simulink model "RobustControl"  (Simulink 7.9)
settings: Solver=ode45  StartTime=0.0  StopTime=10.0  RelTol=1e-3
undefined symbols (not defined in the file): e, kd1, kd2, kd3, kd4, kd5, kd6, kp1, kp2, kp3, kp4, kp5, kp6, LinePTs2Rpm, PosSourceSelect, r, Ts
libraries: powerlib_extras x3
settings Model: Creator=Administrator  LastModifiedBy=Administrator

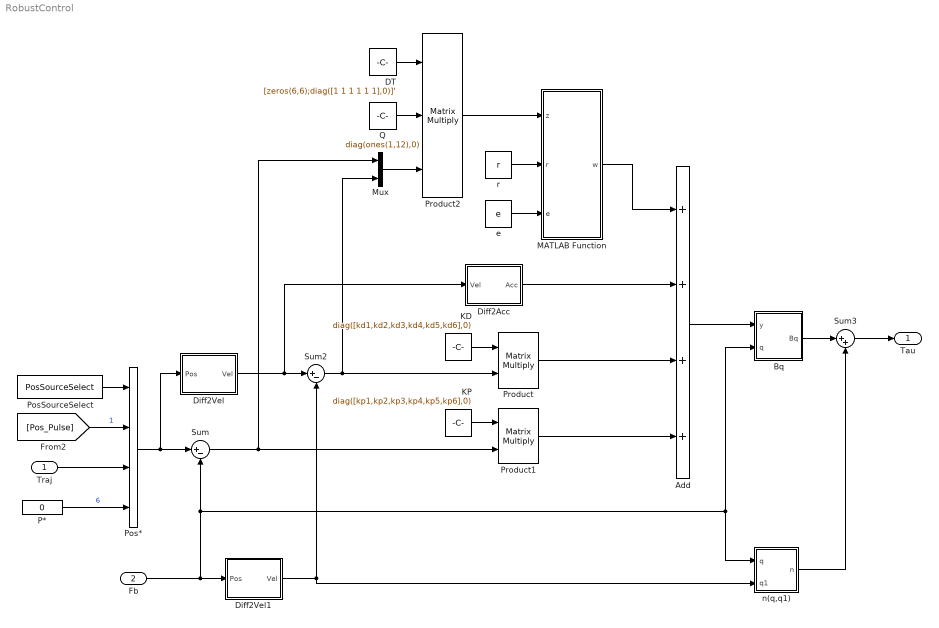
== system RobustControl ==
  Traj : Inport
  Fb : Inport  Port=2
  Add : Sum  Inputs=++++
  Bq : Subsystem
  DT : Constant  Value=[zeros(6,6);diag([1 1 1 1 1 1],0)]'
  Diff2Acc : Subsystem
  Diff2Vel : Subsystem
  Diff2Vel1 : Subsystem
  KD : Constant  Value=diag([kd1,kd2,kd3,kd4,kd5,kd6],0)
  KP : Constant  Value=diag([kp1,kp2,kp3,kp4,kp5,kp6],0)
  MATLAB Function : MATLAB Function  TreatAsAtomicUnit=on
  Mux : Mux  Inputs=2
  P* : Constant  Value=0  SampleTime=Ts
  Pos* : MultiPortSwitch  zeroidx=off  SampleTime=Ts
  PosSourceSelect : Constant  Value=PosSourceSelect  SampleTime=Ts
  Product : Product  Multiplication=Matrix(*)  RndMeth=Zero
  Product1 : Product  Multiplication=Matrix(*)  RndMeth=Zero
  Product2 : Product  Inputs=3  Multiplication=Matrix(*)  RndMeth=Zero
  Q : Constant  Value=diag(ones(1,12),0)
  Sum : Sum  Inputs=|+-  SampleTime=Ts
  Sum2 : Sum  Inputs=|+-  SampleTime=Ts
  Sum3 : Sum  Inputs=|++  SampleTime=Ts
  e : Constant  Value=e
  n(q,q1) : Subsystem
  r : Constant  Value=r
  Tau : Outport
  wires:
  [Pos_Pulse] -> Pos*/2  "1"
  P*/1 -> Pos*/4  "6"
  PosSourceSelect/1 -> Pos*/1
  Diff2Vel/1(Vel) -> Sum2/1, Diff2Acc/1(Vel)
  Diff2Vel1/1(Vel) -> Sum2/2, n(q,q1)/2(q1)
  Bq/1(Bq) -> Sum3/1
  n(q,q1)/1(n) -> Sum3/2
  Sum3/1 -> Tau/1
  Traj/1 -> Pos*/3
  Sum/1 -> Product1/2, Mux/1
  Sum2/1 -> Product/2, Mux/2
  KD/1 -> Product/1
  KP/1 -> Product1/1
  Pos*/1 -> Sum/1, Diff2Vel/1(Pos)
  Fb/1 -> Diff2Vel1/1(Pos), Sum/2, Bq/2(q), n(q,q1)/1(q)
  DT/1 -> Product2/1
  Q/1 -> Product2/2
  Mux/1 -> Product2/3
  Product2/1 -> MATLAB Function/1(z)
  r/1 -> MATLAB Function/2(r)
  e/1 -> MATLAB Function/3(e)
  Add/1 -> Bq/1(y)
  Diff2Acc/1(Acc) -> Add/2
  Product/1 -> Add/3
  Product1/1 -> Add/4
  MATLAB Function/1(w) -> Add/1

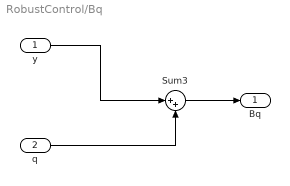
== system RobustControl/Bq ==
  y : Inport
  q : Inport  Port=2
  Sum3 : Sum  Inputs=|++
  Bq : Outport
  wires:
  q/1 -> Sum3/2
  y/1 -> Sum3/1
  Sum3/1 -> Bq/1

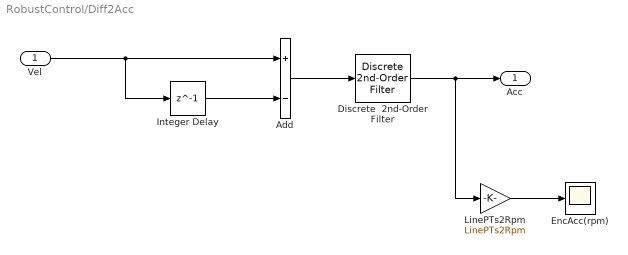
== system RobustControl/Diff2Acc ==
  Vel : Inport
  Add : Sum  Inputs=+-
  Discrete  2nd-Order Filter : powerlib_extras/Discrete  Control Blocks/Discrete  2nd-Order Filter  FilterType=Lowpass  Fo=200  Zeta=0.707  Ts=Ts  Initialize=off  Vac_Init=[0.8 -25 60]  Vdc_Init=-0.4  PlotResponse=off  param1=[1 5000 10]
  EncAcc(rpm) : Scope
      settings: SaveName=ScopeData33
  Integer Delay : Delay  DelayLength=1  InputProcessing=Inherited
  LinePTs2Rpm : Gain  Gain=LinePTs2Rpm
  Acc : Outport
  wires:
  Add/1 -> Discrete  2nd-Order Filter/1
  Discrete  2nd-Order Filter/1 -> Acc/1, LinePTs2Rpm/1
  Vel/1 -> Integer Delay/1, Add/1
  Integer Delay/1 -> Add/2
  LinePTs2Rpm/1 -> EncAcc(rpm)/1

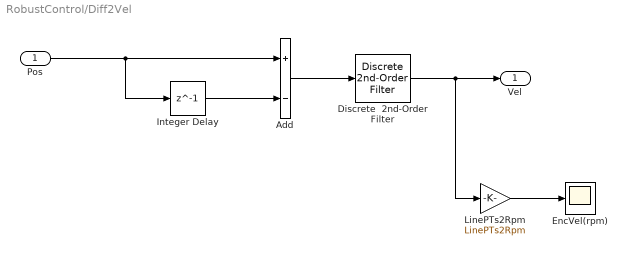
== system RobustControl/Diff2Vel ==
  Pos : Inport
  Add : Sum  Inputs=+-
  Discrete  2nd-Order Filter : powerlib_extras/Discrete  Control Blocks/Discrete  2nd-Order Filter  FilterType=Lowpass  Fo=200  Zeta=0.707  Ts=Ts  Initialize=off  Vac_Init=[0.8 -25 60]  Vdc_Init=-0.4  PlotResponse=off  param1=[1 5000 10]
  EncVel(rpm) : Scope
      settings: SaveName=ScopeData33
  Integer Delay : Delay  DelayLength=1  InputProcessing=Inherited
  LinePTs2Rpm : Gain  Gain=LinePTs2Rpm
  Vel : Outport
  wires:
  Add/1 -> Discrete  2nd-Order Filter/1
  Discrete  2nd-Order Filter/1 -> Vel/1, LinePTs2Rpm/1
  Pos/1 -> Integer Delay/1, Add/1
  Integer Delay/1 -> Add/2
  LinePTs2Rpm/1 -> EncVel(rpm)/1

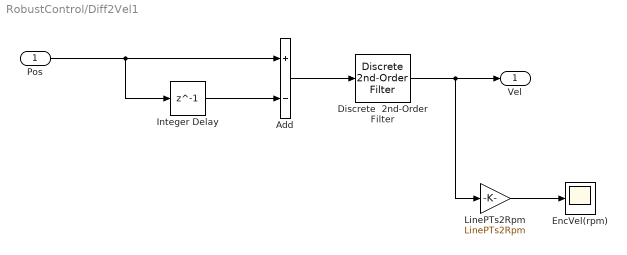
== system RobustControl/Diff2Vel1 ==
  Pos : Inport
  Add : Sum  Inputs=+-
  Discrete  2nd-Order Filter : powerlib_extras/Discrete  Control Blocks/Discrete  2nd-Order Filter  FilterType=Lowpass  Fo=200  Zeta=0.707  Ts=Ts  Initialize=off  Vac_Init=[0.8 -25 60]  Vdc_Init=-0.4  PlotResponse=off  param1=[1 5000 10]
  EncVel(rpm) : Scope
      settings: SaveName=ScopeData33
  Integer Delay : Delay  DelayLength=1  InputProcessing=Inherited
  LinePTs2Rpm : Gain  Gain=LinePTs2Rpm
  Vel : Outport
  wires:
  Add/1 -> Discrete  2nd-Order Filter/1
  Discrete  2nd-Order Filter/1 -> Vel/1, LinePTs2Rpm/1
  Pos/1 -> Integer Delay/1, Add/1
  Integer Delay/1 -> Add/2
  LinePTs2Rpm/1 -> EncVel(rpm)/1

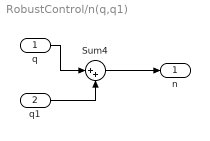
== system RobustControl/n(q,q1) ==
  q : Inport
  q1 : Inport  Port=2
  Sum4 : Sum  Inputs=|++  SampleTime=Ts
  n : Outport
  wires:
  Sum4/1 -> n/1
  q/1 -> Sum4/1
  q1/1 -> Sum4/2

== matlab function MATLAB Function ==
  data: z input double; r input double; w output double; e input double
function w= fcn(z,r,e)
%#codegen
if norm(z)>=e
    w=(r/norm(z))*z;
else
    w=(r/e)*z;
end
end
